simulink library "configurationExampleLibrary"  (R2019a)
settings: Solver=VariableStepAuto  StartTime=0.0  StopTime=10.0  RelTol=1e-3
settings Model: Creator=jnicholson  LastModifiedBy=jnicholson

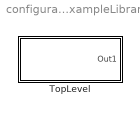
== system configurationExampleLibrary ==
  TopLevel : Subsystem  mask{optionA=6, optionB=2, isOptionCenabled=off, optionC=0, optionD=60, optionE=22, optionF=none}
      mask prompts: optionA "Option A"; optionB "Option B"; isOptionCenabled "Enable Option C"; optionC "Option C"; optionD "Option D"; optionE "Option E"; optionF "Option F"
      mask init:
      | topLevel_Initialization % run initialization script
      mask TypeOptions optionA: 1 | 2 | 3 | 4 | 5 | 6
      mask Callback optionA: optionA_callback(gcbh)
      mask TypeOptions optionB: 1 | 2
      mask Callback optionB: optionB_callback(gcbh)
      mask Callback isOptionCenabled: optionCisEnabled_callback(gcbh)
      mask TypeOptions optionD: 37 | 38 | 39 | 40 | 41 | 42 | 43 | 44 | 56 | 57 | 59 | 60
      mask Callback optionD: optionD_callback(gcbh)
      mask TypeOptions optionE: 1 | 2 | 3 | 4 | 5 | 6 | 7 | 8 | 9 | 10 | 11 | 12 | 13 | 14 | 15 | 16 | 17 | 18 | 19 | 20 | 21 | 22
      mask TypeOptions optionF: none

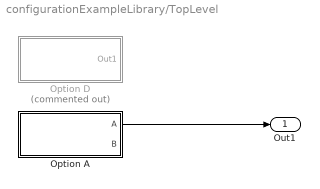
== system configurationExampleLibrary/TopLevel ==
  Option A : Subsystem  VariantControlMode=Label  Variant=on  LabelModeActiveChoice=Option_6
  Option D : Subsystem  Commented=on  Variant=on
  Out1 : Outport
  wires:
  Option A/1(A) -> Out1/1

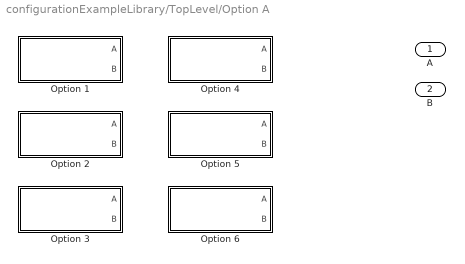
== system configurationExampleLibrary/TopLevel/Option A ==
  Option 1 : Subsystem  VariantControl=Option_1  mask{optionB=2, optionC=0}
      mask prompts: optionB "Option B"; optionC "Option C"
      mask Display: fprintf('optionB = %s', optionB);
  Option 2 : Subsystem  VariantControl=Option_2  mask{optionB=1}
      mask prompts: optionB "Option B"
      mask Display: fprintf('optionB = %s', optionB);
  Option 3 : Subsystem  VariantControl=Option_3  mask{optionB=5}
      mask prompts: optionB "Option B"
      mask Display: fprintf('optionB = %s', optionB);
  Option 4 : Subsystem  VariantControl=Option_4  mask{optionB=2}
      mask prompts: optionB "Option B"
      mask Display: fprintf('optionB = %s', optionB);
  Option 5 : Subsystem  VariantControl=Option_5  mask{optionB=3}
      mask prompts: optionB "Option B"
      mask Display: fprintf('optionB = %s', optionB);
  Option 6 : Subsystem  VariantControl=Option_6  mask{optionB=2}
      mask prompts: optionB "Option B"
      mask Display: fprintf('optionB = %s', optionB);
  A : Outport
  B : Outport  Port=2

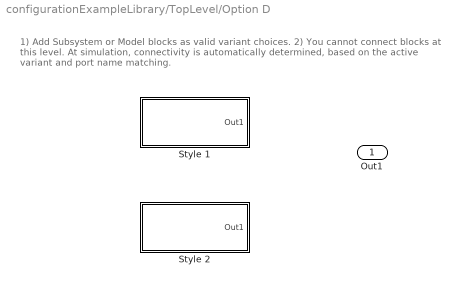
== system configurationExampleLibrary/TopLevel/Option D ==
  note: 1) Add Subsystem or Model blocks as valid variant choices.
      | 2) You cannot connect blocks at this level. At simulation, connectivity is automatically
      | determined, based on the active variant and port name matching.
  Style 1 : Subsystem  VariantControl=Choice_1
  Style 2 : Subsystem  VariantControl=Choice_2
  Out1 : Outport

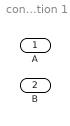
== system configurationExampleLibrary/TopLevel/Option A/Option 1 ==
  A : Outport
  B : Outport  Port=2

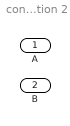
== system configurationExampleLibrary/TopLevel/Option A/Option 2 ==
  A : Outport
  B : Outport  Port=2

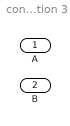
== system configurationExampleLibrary/TopLevel/Option A/Option 3 ==
  A : Outport
  B : Outport  Port=2

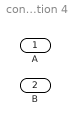
== system configurationExampleLibrary/TopLevel/Option A/Option 4 ==
  A : Outport
  B : Outport  Port=2

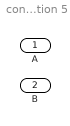
== system configurationExampleLibrary/TopLevel/Option A/Option 5 ==
  A : Outport
  B : Outport  Port=2

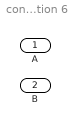
== system configurationExampleLibrary/TopLevel/Option A/Option 6 ==
  A : Outport
  B : Outport  Port=2

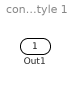
== system configurationExampleLibrary/TopLevel/Option D/Style 1 ==
  Out1 : Outport

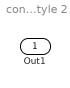
== system configurationExampleLibrary/TopLevel/Option D/Style 2 ==
  Out1 : Outport
